simulink model "synth_fir_tb"  (Simulink 7.1)
settings: Solver=ode45  StartTime=0.0  StopTime=160  RelTol=1e-3
undefined symbols (not defined in the file or in its folder): mem
libraries: xbsIndex_r4 x80, xbsCopyrightNotice_r4 x1, dspsigops x1, dspsrcs4 x1
settings Model: Creator=alexc  LastModifiedBy=thuyp
settings DataIOCC: SignalLoggingName=sigsOut
settings OptimizationCC: InlineInvariantSignals=on
settings DebuggingCC: SaveWithParameterizedLinksMsg=none  SignalResolutionControl=TryResolveAllWithWarning  SolverPrmCheckMsg=none  MultiTaskDSMMsg=warning  MultiTaskCondExecSysMsg=none  StrictBusMsg=None
settings HardwareCC: TargetUnknown=on
settings RTWCC: IncludeERTFirstTime=on
settings GRTTargetCC: TargetFcnLib=ansi_tfl_tmw.mat

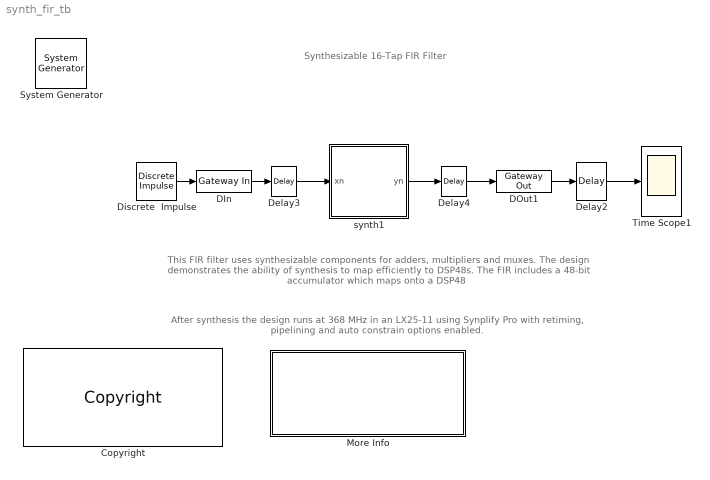
== system synth_fir_tb ==
  note: Synthesizable 16-Tap FIR Filter
  note: This FIR filter uses synthesizable components
      | for adders, multipliers and muxes. The design demonstrates
      |  the ability of synthesis to map efficiently to DSP48s.
      | The FIR includes a 48-bit accumulator which maps onto a DSP48
  note: After synthesis the design runs at 368 MHz in an LX25-11
      | using Synplify Pro with retiming, pipelining and auto constrain options enabled.
  " System Generator" : xbsIndex_r4/ System Generator  Tag=genX  SystemSampleTime=-1  xilinxfamily=virtex4  part=xc4vsx35  speed=-10  package=ff668  synthesis_tool=XST  clock_wrapper=Clock Enables  directory=./netlist  testbench=off  simulink_period=1  sysclk_period=2.90  dcm_input_clock_period=100  incr_netlist=off  trim_vbits=Everywhere in SubSystem  dbl_ovrd=According to Block Masks  core_generation=According to Block Masks  run_coregen=off  deprecated_control=off  eval_field=0  block_type=system_generator
      settings: block_version=8.2.EA1
  Copyright : xbsCopyrightNotice_r4/Copyright  copyrighttext="Copyright (c) 2009  by  Xilinx, Inc. All rights reserved.<br><br>This file contains proprietary, confidential information of Xilinx, Inc., is distributed under licensefrom Xilinx, Inc., and may be used, copied and/or disclosed only pursuant to the terms of a valid licenseagreement with Xilinx, Inc. Xilinx hereby grants you a license to use this file solely for design,simulation, implementation and creation of design files limited to Xilinx devices or technologies. Use with non-Xilinx devices or technologies is expressly prohibited and immediately terminates your license unless covered by a separate agreement.<br><br>Xilinx is providing this design, code, or information \"as-is\" solely for use in developing programs and solutions for Xilinx devices, with no obligation on the part of Xilinx to provide support. By providingthis design, code, or information as one possible implementation of this feature, application or standard,Xilinx is making no representation that this implementation is free from any claims of infringement. Youare responsible for obtaining any rights you may require for your implementation. Xilinx expressly disclaimsany warranty whatsoever with respect to the adequacy of the implementation, including but not limited to anywarranties or representations that this implementation is free from claims of infringement, implied warrantiesof merchantability or fitness for a particular purpose.<br><br>Xilinx products are not intended for use in life support appliances, devices, or systems. Use in such applications is expressly prohibited.<br><br>Any modifications that are made to the Source Code are done at the user's sole risk and will be unsupported.<br><br>This copyright and support notice must be retained as part of this text at all times. (c) Copyright 1995-2009 Xilinx, Inc. All rights reserved."  block_type=copyright
      settings: block_version=10.1.00
      settings: infoedit=|
      | Copyright(C) 2008 by  Xilinx, Inc. All rights reserved.<br>
      | <br>
      | This file contains proprietary, confidential information of Xilinx, Inc., is distributed under license
      | from Xilinx, Inc., and may be used, copied and/or disclosed only pursuant to the terms of a valid license
      | agreement with Xilinx, Inc. Xilinx hereby grants you a license to use this file solely for design,
      | simulation, implementation and creation of design files limited to Xilinx devices or technologies. Use
      | with non-Xilinx devices or technologies is expressly prohibited and immediately terminates your license
      | unless covered by a separate agreement.<br>
      | <br>
      | Xilinx is providing this design, code, or information "as-is" solely for use in developing programs and
      | solutions for Xilinx devices, with no obligation on the part of Xilinx to provide support. By providing
      | this design, code, or information as one possible implementation of this feature, application or standard,
      | Xilinx is making no representation that this implementation is free from any claims of infringement. You
      | are responsible for obtaining any rights you may require for your implementation. Xilinx expressly disclaims
      | any warranty whatsoever with respect to the adequacy of the implementation, including but not limited to any
      | warranties or representations that this implementation is free from claims of infringement, implied warranties
      | of merchantability or fitness for a particular purpose.<br>
      | <br>
      | Xilinx products are not intended for use in life support appliances, devices, or systems. Use in such
      | applications is expressly prohibited.<br>
      | <br>
      | Any modifications that are made to the Source Code are done at the user's sole risk and will be unsupported.<br>
      | <br>
      | This copyright and support notice must be retained as part of this text at all times.
      | (c) Copyright 1995-2008 Xilinx, Inc. All rights reserved.
  DIn : xbsIndex_r4/Gateway In  arith_type="Signed  (2's comp)"  n_bits=18  bin_pt=0  quantization="Round  (unbiased: +/- Inf)"  overflow=Saturate  period=4  dbl_ovrd=off  timing_constraint=None  locs_specified=off  LOCs={}  block_type=gatewayin
      settings: infoedit="Gateway in block.  Converts inputs of type Simulink integer, double and fixed point to  Xilinx fixed point type.<P><P>Hardware notes:  In hardware these blocks become top level input ports."  xl_area=[0 0 0 0 18 0 0]  block_version=VER_STRING_GOES_HERE
  DOut1 : xbsIndex_r4/Gateway Out  hdl_port=on  timing_constraint=None  locs_specified=off  LOCs={}  block_type=gatewayout
      settings: infoedit="Gateway out block.  Converts Xilinx fixed point inputs into ouputs of type Simulink integer, double, or fixed point.<P><P>Hardware notes:  In hardware these blocks become top level output ports or are discarded, depending on how they are configured."  xl_area=[0 0 0 0 48 0 0]  block_version=VER_STRING_GOES_HERE
  Delay2 : dspsigops/Delay  dly_unit=Samples  delay=1  ic_detail=off  dif_ic_for_ch=off  dif_ic_for_dly=off  ic=0  reset_popup=None
  Delay3 : xbsIndex_r4/Delay  en=off  latency=3  dbl_ovrd=off  reg_retiming=on  block_type=delay
      settings: infoedit="Delay line having  configurable length.<P><P>Hardware notes: A delay line is a chain, each link of which is an SRL16 followed by a flip-flop. If register retiming is enabled, the delay line is a chain of flip-flops."  xl_area=[0, 0, 0, 0, 0, 0, 0]  block_version=VER_STRING_GOES_HERE
  Delay4 : xbsIndex_r4/Delay  en=off  latency=3  dbl_ovrd=off  reg_retiming=on  block_type=delay
      settings: infoedit="Delay line having  configurable length.<P><P>Hardware notes: A delay line is a chain, each link of which is an SRL16 followed by a flip-flop. If register retiming is enabled, the delay line is a chain of flip-flops."  xl_area=[0, 0, 0, 0, 0, 0, 0]  block_version=VER_STRING_GOES_HERE
  Discrete  Impulse : dspsrcs4/Discrete  Impulse  Delay=0  SampleTime=4  FrameSample=1  dataType=double  isSigned=on  wordLen=16  udDataType=sfix(16)  fracBitsMode=Best precision  numFracBits=15
  More Info : Subsystem
      settings: OpenFcn=xlDoc('-book','sysgen','-topic','Hardware Design Using System Generator/Design Styles for the DSP48/Designs that Use DSP48 and DSP48 Macro Blocks');
      mask Display: disp('Double click\n for System Generator\n documentation on related topics.')
  Time Scope1 : Scope
      settings: DataFormat=Structure
  synth1 : Subsystem  mask{bit_width=18, bin_pt=0, coef=fir1(15,0.3), coef_bit_width=18, coef_bin_pt=18, m=4, Ts=4}
      mask prompts: bit_width "Input Data Width"; bin_pt "Input Data Binary Point"; coef "Coefficients"; coef_bit_width "Coefficient Bit Width"; coef_bin_pt "Coefficient Binary Point"; m "Number of Multipliers"; Ts "Sample Period"
      mask init:
      | %accounts for the pull down GUI value
      | 
      | no_mults = 4; % for this implementation
      | 
      | %pad the coefficients to be a multiple of the interp_ratio*no_mults
      | multiple_test = ((ceil(length(coef)/no_mults)) - (length(coef)/no_mults)) * no_mults;
      | if (multiple_test > 0)
      | 	coef = [coef(:)' zeros(1,multiple_test)];
      | end
      | 
      | no_taps = length(coef);
      | taps_per_mult = no_taps/no_mults;
      |     
      | %form DRAM values
      | z = zeros(1,taps_per_mult);
      | 
      | for k = 0:(no_mults-1)
      |     for p = 0:(taps_per_mult-1)
      |         mem(p+1,k+1) = coef((k*4)+p+1);
      |     end
      | end
      | 
      | x_SRL_depth = taps_per_mult;
      | upsamp_by = x_SRL_depth;
      | downsamp_by = taps_per_mult;
      | T_clock = Ts/upsamp_by;
      | bit_growth = 2 + ceil(log2(x_SRL_depth));
      | y_bit_width = bit_width + coef_bit_width + bit_growth;
      | 
      | %Display graphic on the block
      | dstr1 = sprintf('%d tap', no_taps);
      | 
      | [bg,fg] = xlcmap('XBlock',0);
      | iPos = get_param(gcb,'Position');
      | iWidth=iPos(3)-iPos(1); iHeight=iPos(4)-iPos(2);
      | iCx=iWidth/2;
      | iCy=iHeight/2;
      | [logoX, logoY] = xlogo(iPos);
      mask StyleString: edit,edit,edit,edit,edit,popup(1|2|3|4|5|6|7|8|9|10|11|12|13|14|15|16|17|18|19|20|21|22|23|24),edit
      mask Display:
      | patch([0 iWidth iWidth 0],[0 0 iHeight iHeight] , bg);
      | patch(logoX,logoY, fg);
      | text(iCx/1.3,iCy+15,dstr1);
      | text(iCx/1.5-4,iCy-5,'MAC FIR');
      | plot([0 0 iWidth iWidth 0], [0 iHeight iHeight 0 0]);
  wires:
  DIn/1 -> Delay3/1
  Discrete  Impulse/1 -> DIn/1
  DOut1/1 -> Delay2/1
  Delay2/1 -> Time Scope1/1
  synth1/1(yn) -> Delay4/1
  Delay3/1 -> synth1/1(xn)
  Delay4/1 -> DOut1/1

== system synth_fir_tb/More Info ==

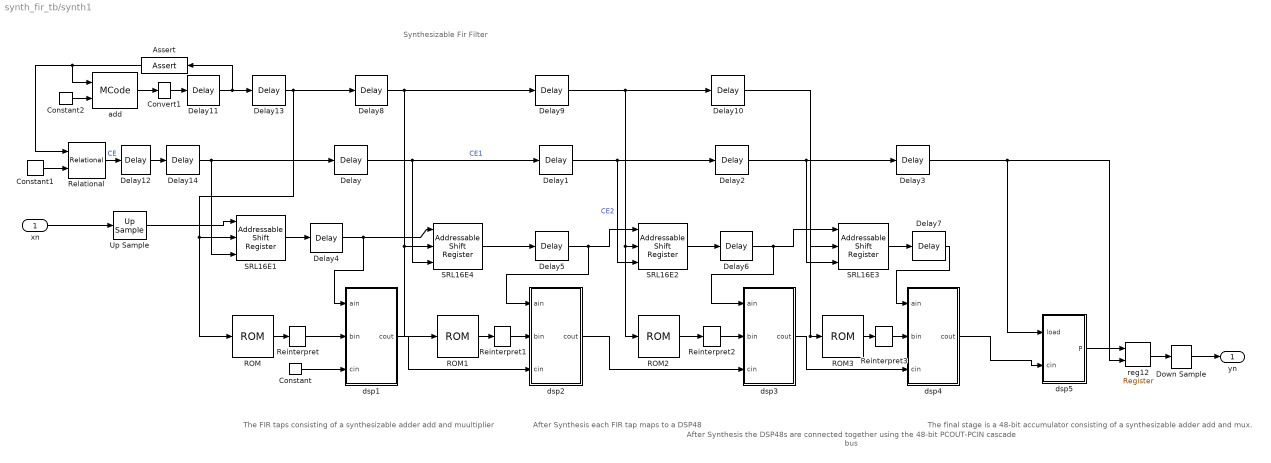
== system synth_fir_tb/synth1 ==
  note: The final stage is a 48-bit accumulator consisting of a
      | synthesizable adder add and mux.
  note: The FIR taps consisting of a
      | synthesizable adder add and muultiplier
  note: After Synthesis each FIR tap maps to a DSP48
  note: After Synthesis the DSP48s are connected together
      | using the 48-bit PCOUT-PCIN cascade bus
  note: Synthesizable Fir Filter
  xn : Inport  OutDataType=sfix(16)  OutScaling=2^0
  Assert : xbsIndex_r4/Assert  Orientation=left  assert_type=off  type_source=Explicitly  arith_type=Unsigned  n_bits=8  bin_pt=2  assert_rate=on  rate_source=Explicitly  period=1  output_port=on  block_type=assert
      settings: infoedit=Asserts a user-defined sample rate and/or type on a signal.  block_version=VER_STRING_GOES_HERE
  Constant : xbsIndex_r4/Constant  arith_type=Signed (2's comp)  const=0  n_bits=48  bin_pt=0  explicit_period=off  period=1  equ=P=C  opselect=C  inp2=PCIN>>17  opr=+  inp1=P  carry=CIN  dbl_ovrd=off  block_type=constant
      settings: block_version=VER_STRING_GOES_HERE
  Constant1 : xbsIndex_r4/Constant  arith_type=Unsigned  const=2  n_bits=2  bin_pt=0  explicit_period=off  period=1  equ=P=C  opselect=C  inp2=PCIN>>17  opr=+  inp1=P  carry=CIN  dbl_ovrd=off  block_type=constant
      settings: block_version=VER_STRING_GOES_HERE
  Constant2 : xbsIndex_r4/Constant  arith_type=Unsigned  const=1  n_bits=2  bin_pt=0  explicit_period=off  period=1  equ=P=C  opselect=C  inp2=PCIN>>17  opr=+  inp1=P  carry=CIN  dbl_ovrd=off  block_type=constant
      settings: block_version=VER_STRING_GOES_HERE
  Convert1 : xbsIndex_r4/Convert  arith_type=Unsigned  n_bits=2  bin_pt=0  quantization=Truncate  overflow=Wrap  latency=0  dbl_ovrd=off  pipeline=off  block_type=convert
      settings: infoedit=The input is presented at the output after quantization and overflow effects.<P><P>Hardware notes: Additional hardware is used when rounding or saturation is selected and output width is less than the input width.  xl_area=[0, 0, 0, 0, 0, 0, 0]  block_version=VER_STRING_GOES_HERE
  Delay{,1..14} (15 alike) : xbsIndex_r4/Delay  en=off  latency=1  dbl_ovrd=off  reg_retiming=on  block_type=delay
      settings: infoedit="Delay line having  configurable length.<P><P>Hardware notes: A delay line is a chain, each link of which is an SRL16 followed by a flip-flop. If register retiming is enabled, the delay line is a chain of flip-flops."  xl_area=[0, 0, 0, 0, 0, 0, 0]  block_version=VER_STRING_GOES_HERE
  Down Sample : xbsIndex_r4/Down Sample  sample_ratio=4  sample_phase="Last Value of Frame  (most efficient)"  en=off  latency=1  dbl_ovrd=off  block_type=dsamp
      settings: xl_area=[24 48 0 0 0 0 0]  block_version=VER_STRING_GOES_HERE
  ROM : xbsIndex_r4/ROM  depth=taps_per_mult  initVector=mem(:,1)  distributed_mem=Distributed memory  rst=off  init_reg=0  en=off  latency=1  arith_type="Signed  (2's comp)"  n_bits=coef_bit_width  bin_pt=coef_bin_pt  dbl_ovrd=off  optimize=Area  use_rpm=off  block_type=sprom
      settings: xl_area=[18 18 0 18 0 0 0]  block_version=VER_STRING_GOES_HERE
  ROM1 : xbsIndex_r4/ROM  depth=taps_per_mult  initVector=mem(:,2)  distributed_mem=Distributed memory  rst=off  init_reg=0  en=off  latency=1  arith_type="Signed  (2's comp)"  n_bits=coef_bit_width  bin_pt=coef_bin_pt  dbl_ovrd=off  optimize=Area  use_rpm=off  block_type=sprom
      settings: xl_area=[18 18 0 17 0 0 0]  block_version=VER_STRING_GOES_HERE
  ROM2 : xbsIndex_r4/ROM  depth=taps_per_mult  initVector=mem(:,3)  distributed_mem=Distributed memory  rst=off  init_reg=0  en=off  latency=1  arith_type="Signed  (2's comp)"  n_bits=coef_bit_width  bin_pt=coef_bin_pt  dbl_ovrd=off  optimize=Area  use_rpm=off  block_type=sprom
      settings: xl_area=[18 18 0 17 0 0 0]  block_version=VER_STRING_GOES_HERE
  ROM3 : xbsIndex_r4/ROM  depth=taps_per_mult  initVector=mem(:,4)  distributed_mem=Distributed memory  rst=off  init_reg=0  en=off  latency=1  arith_type="Signed  (2's comp)"  n_bits=coef_bit_width  bin_pt=coef_bin_pt  dbl_ovrd=off  optimize=Area  use_rpm=off  block_type=sprom
      settings: xl_area=[18 18 0 18 0 0 0]  block_version=VER_STRING_GOES_HERE
  Reinterpret{,1..3} (4 alike) : xbsIndex_r4/Reinterpret  force_arith_type=on  arith_type="Signed  (2's comp)"  force_bin_pt=on  bin_pt=0  block_type=cast
      settings: infoedit="Changes type of samples without altering their binary representation.<P><P>Hardware notes: In hardware this block costs nothing.<P><P>Example:  Suppose the input is 6 bits wide, signed, with 2 fractional bits, and the output is forced to unsigned with 0 fractional bits.  Then an input of -2.0 (1110.00 in binary 2's complement) becomes an output of 56 (111000 in binary)."  block_version=VER_STRING_GOES_HERE
  Relational : xbsIndex_r4/Relational  mode=a=b  en=off  latency=0  dbl_ovrd=off  block_type=relational
      settings: xl_area=[1 0 0 1 0 0 0]  block_version=VER_STRING_GOES_HERE
  SRL16E{1..4} (4 alike) : xbsIndex_r4/Addressable Shift Register  infer_latency=off  depth=x_SRL_depth  initVector=[0]  en=on  dbl_ovrd=off  use_behavioral_HDL=off  use_rpm=off  block_type=addrsr
      settings: infoedit="Delay of configurable length.  Any element in the delay line can be addressed and driven onto the output port.<P><P>Hardware notes: Implemented using SRL16s.  If a Virtex-II device is used, multiple SRLC16s are cascaded together."  xl_area=[9 0 0 18 0 0 0]  block_version=VER_STRING_GOES_HERE
  Up Sample : xbsIndex_r4/Up Sample  sample_ratio=taps_per_mult  copy_samples=on  dbl_ovrd=off  block_type=usamp
      settings: infoedit="Up samples input data.  Inserted values  can be zeros or copies of the most recent input sample.<P><P>Hardware notes: No hardware is needed if inserted values are copies of the input sample; otherwise, a mux and single bit flip-flop are used."  xl_area=[0 0 0 0 0 0 0]  block_version=VER_STRING_GOES_HERE
  add : xbsIndex_r4/MCode  mfname=xlsynadd  explicit_period=off  period=1  dbl_ovrd=off  enable_stdout=off  enable_debug=off  suppress_output=off  defparams={}  hide_port_list={}  block_type=mcode
      settings: xl_area=[0, 0, 0, 0, 0, 0, 0]  block_version=8.1
  dsp1 : Subsystem
  dsp2 : Subsystem
  dsp3 : Subsystem
  dsp4 : Subsystem
  dsp5 : Subsystem
  reg12 : xbsIndex_r4/Register  init=0  rst=off  en=on  dbl_ovrd=off  block_type=register
      settings: xl_area=[24 48 0 0 0 0 0]  block_version=VER_STRING_GOES_HERE
  yn : Outport  OutDataType=sfix(16)  OutScaling=2^0
  wires:
  dsp4/1(cout) -> dsp5/2(cin)
  Convert1/1 -> Delay11/1
  Delay11/1 -> Delay13/1, Assert/1
  add/1 -> Convert1/1
  Constant2/1 -> add/2
  Reinterpret3/1 -> dsp4/2(bin)
  Reinterpret2/1 -> dsp3/2(bin)
  Reinterpret1/1 -> dsp2/2(bin)
  Reinterpret/1 -> dsp1/2(bin)
  ROM/1 -> Reinterpret/1
  Constant/1 -> dsp1/3(cin)
  SRL16E1/1 -> Delay4/1
  SRL16E4/1 -> Delay5/1
  dsp1/1(cout) -> dsp2/3(cin)
  ROM1/1 -> Reinterpret1/1
  ROM2/1 -> Reinterpret2/1
  ROM3/1 -> Reinterpret3/1
  dsp2/1(cout) -> dsp3/3(cin)
  dsp3/1(cout) -> dsp4/3(cin)
  SRL16E2/1 -> Delay6/1
  SRL16E3/1 -> Delay7/1
  Delay10/1 -> SRL16E3/2, ROM3/1
  Delay4/1 -> SRL16E4/1, dsp1/1(ain)
  Delay5/1 -> SRL16E2/1, dsp2/1(ain)
  Delay6/1 -> SRL16E3/1, dsp3/1(ain)
  Constant1/1 -> Relational/2
  Relational/1 -> Delay12/1  "CE"
  Delay2/1 -> Delay3/1, SRL16E3/3
  xn/1 -> Up Sample/1
  dsp5/1(P) -> reg12/1
  Up Sample/1 -> SRL16E1/1
  reg12/1 -> Down Sample/1
  Down Sample/1 -> yn/1
  Delay7/1 -> dsp4/1(ain)
  Delay3/1 -> reg12/2, dsp5/1(load)
  Delay12/1 -> Delay14/1
  Delay8/1 -> Delay9/1, SRL16E4/2, ROM1/1
  Delay9/1 -> Delay10/1, SRL16E2/2, ROM2/1
  Delay1/1 -> Delay2/1, SRL16E2/3  "CE2"
  Delay/1 -> Delay1/1, SRL16E4/3  "CE1"
  Delay13/1 -> Delay8/1, ROM/1, SRL16E1/2
  Delay14/1 -> Delay/1, SRL16E1/3
  Assert/1 -> add/1, Relational/1

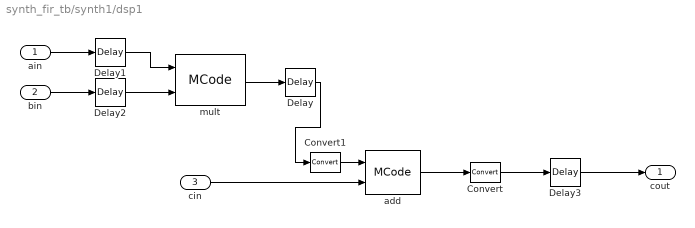
== system synth_fir_tb/synth1/dsp1 ==
  ain : Inport  OutDataType=sfix(16)  OutScaling=2^0
  bin : Inport  Port=2  OutDataType=sfix(16)  OutScaling=2^0
  cin : Inport  Port=3  OutDataType=sfix(16)  OutScaling=2^0
  Convert : xbsIndex_r4/Convert  arith_type="Signed  (2's comp)"  n_bits=48  bin_pt=0  quantization=Truncate  overflow=Wrap  latency=0  dbl_ovrd=off  pipeline=off  block_type=convert
      settings: infoedit=The input is presented at the output after quantization and overflow effects.<P><P>Hardware notes: Additional hardware is used when rounding or saturation is selected and output width is less than the input width.  xl_area=[0, 0, 0, 0, 0, 0, 0]  block_version=VER_STRING_GOES_HERE
  Convert1 : xbsIndex_r4/Convert  arith_type="Signed  (2's comp)"  n_bits=48  bin_pt=0  quantization=Truncate  overflow=Wrap  latency=0  dbl_ovrd=off  pipeline=off  block_type=convert
      settings: infoedit=The input is presented at the output after quantization and overflow effects.<P><P>Hardware notes: Additional hardware is used when rounding or saturation is selected and output width is less than the input width.  xl_area=[0, 0, 0, 0, 0, 0, 0]  block_version=VER_STRING_GOES_HERE
  Delay{,1..3} (4 alike) : xbsIndex_r4/Delay  en=off  latency=1  dbl_ovrd=off  reg_retiming=on  block_type=delay
      settings: infoedit="Delay line having  configurable length.<P><P>Hardware notes: A delay line is a chain, each link of which is an SRL16 followed by a flip-flop. If register retiming is enabled, the delay line is a chain of flip-flops."  xl_area=[0, 0, 0, 0, 0, 0, 0]  block_version=VER_STRING_GOES_HERE
  add : xbsIndex_r4/MCode  mfname=xlsynadd  explicit_period=off  period=1  dbl_ovrd=off  enable_stdout=off  enable_debug=off  suppress_output=off  defparams={}  hide_port_list={}  block_type=mcode
      settings: xl_area=[0, 0, 0, 0, 0, 0, 0]  block_version=8.1
  mult : xbsIndex_r4/MCode  mfname=xlsynmult  explicit_period=off  period=1  dbl_ovrd=off  enable_stdout=off  enable_debug=off  suppress_output=off  defparams={}  hide_port_list={}  block_type=mcode
      settings: xl_area=[0, 0, 0, 0, 0, 0, 0]  block_version=8.1
  cout : Outport  OutDataType=sfix(16)  OutScaling=2^0
  wires:
  Convert1/1 -> add/1
  Convert/1 -> Delay3/1
  Delay/1 -> Convert1/1
  Delay1/1 -> mult/1
  Delay2/1 -> mult/2
  Delay3/1 -> cout/1
  add/1 -> Convert/1
  cin/1 -> add/2
  mult/1 -> Delay/1
  bin/1 -> Delay2/1
  ain/1 -> Delay1/1

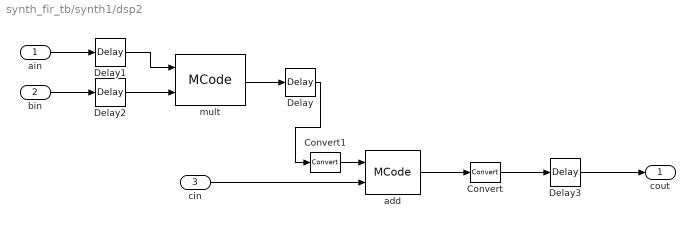
== system synth_fir_tb/synth1/dsp2 ==
  ain : Inport  OutDataType=sfix(16)  OutScaling=2^0
  bin : Inport  Port=2  OutDataType=sfix(16)  OutScaling=2^0
  cin : Inport  Port=3  OutDataType=sfix(16)  OutScaling=2^0
  Convert : xbsIndex_r4/Convert  arith_type="Signed  (2's comp)"  n_bits=48  bin_pt=0  quantization=Truncate  overflow=Wrap  latency=0  dbl_ovrd=off  pipeline=off  block_type=convert
      settings: infoedit=The input is presented at the output after quantization and overflow effects.<P><P>Hardware notes: Additional hardware is used when rounding or saturation is selected and output width is less than the input width.  xl_area=[0, 0, 0, 0, 0, 0, 0]  block_version=VER_STRING_GOES_HERE
  Convert1 : xbsIndex_r4/Convert  arith_type="Signed  (2's comp)"  n_bits=48  bin_pt=0  quantization=Truncate  overflow=Wrap  latency=0  dbl_ovrd=off  pipeline=off  block_type=convert
      settings: infoedit=The input is presented at the output after quantization and overflow effects.<P><P>Hardware notes: Additional hardware is used when rounding or saturation is selected and output width is less than the input width.  xl_area=[0, 0, 0, 0, 0, 0, 0]  block_version=VER_STRING_GOES_HERE
  Delay{,1..3} (4 alike) : xbsIndex_r4/Delay  en=off  latency=1  dbl_ovrd=off  reg_retiming=on  block_type=delay
      settings: infoedit="Delay line having  configurable length.<P><P>Hardware notes: A delay line is a chain, each link of which is an SRL16 followed by a flip-flop. If register retiming is enabled, the delay line is a chain of flip-flops."  xl_area=[0, 0, 0, 0, 0, 0, 0]  block_version=VER_STRING_GOES_HERE
  add : xbsIndex_r4/MCode  mfname=xlsynadd  explicit_period=off  period=1  dbl_ovrd=off  enable_stdout=off  enable_debug=off  suppress_output=off  defparams={}  hide_port_list={}  block_type=mcode
      settings: xl_area=[0, 0, 0, 0, 0, 0, 0]  block_version=8.1
  mult : xbsIndex_r4/MCode  mfname=xlsynmult  explicit_period=off  period=1  dbl_ovrd=off  enable_stdout=off  enable_debug=off  suppress_output=off  defparams={}  hide_port_list={}  block_type=mcode
      settings: xl_area=[0, 0, 0, 0, 0, 0, 0]  block_version=8.1
  cout : Outport  OutDataType=sfix(16)  OutScaling=2^0
  wires:
  ain/1 -> Delay1/1
  bin/1 -> Delay2/1
  mult/1 -> Delay/1
  cin/1 -> add/2
  add/1 -> Convert/1
  Delay3/1 -> cout/1
  Delay2/1 -> mult/2
  Delay1/1 -> mult/1
  Delay/1 -> Convert1/1
  Convert/1 -> Delay3/1
  Convert1/1 -> add/1

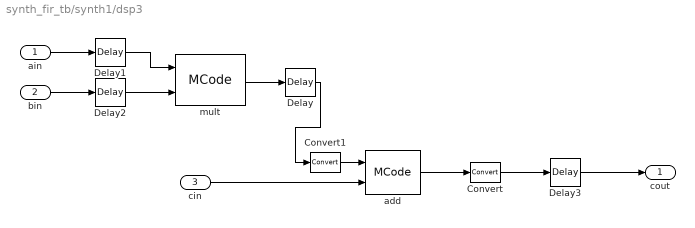
== system synth_fir_tb/synth1/dsp3 ==
  ain : Inport  OutDataType=sfix(16)  OutScaling=2^0
  bin : Inport  Port=2  OutDataType=sfix(16)  OutScaling=2^0
  cin : Inport  Port=3  OutDataType=sfix(16)  OutScaling=2^0
  Convert : xbsIndex_r4/Convert  arith_type="Signed  (2's comp)"  n_bits=48  bin_pt=0  quantization=Truncate  overflow=Wrap  latency=0  dbl_ovrd=off  pipeline=off  block_type=convert
      settings: infoedit=The input is presented at the output after quantization and overflow effects.<P><P>Hardware notes: Additional hardware is used when rounding or saturation is selected and output width is less than the input width.  xl_area=[0, 0, 0, 0, 0, 0, 0]  block_version=VER_STRING_GOES_HERE
  Convert1 : xbsIndex_r4/Convert  arith_type="Signed  (2's comp)"  n_bits=48  bin_pt=0  quantization=Truncate  overflow=Wrap  latency=0  dbl_ovrd=off  pipeline=off  block_type=convert
      settings: infoedit=The input is presented at the output after quantization and overflow effects.<P><P>Hardware notes: Additional hardware is used when rounding or saturation is selected and output width is less than the input width.  xl_area=[0, 0, 0, 0, 0, 0, 0]  block_version=VER_STRING_GOES_HERE
  Delay{,1..3} (4 alike) : xbsIndex_r4/Delay  en=off  latency=1  dbl_ovrd=off  reg_retiming=on  block_type=delay
      settings: infoedit="Delay line having  configurable length.<P><P>Hardware notes: A delay line is a chain, each link of which is an SRL16 followed by a flip-flop. If register retiming is enabled, the delay line is a chain of flip-flops."  xl_area=[0, 0, 0, 0, 0, 0, 0]  block_version=VER_STRING_GOES_HERE
  add : xbsIndex_r4/MCode  mfname=xlsynadd  explicit_period=off  period=1  dbl_ovrd=off  enable_stdout=off  enable_debug=off  suppress_output=off  defparams={}  hide_port_list={}  block_type=mcode
      settings: xl_area=[0, 0, 0, 0, 0, 0, 0]  block_version=8.1
  mult : xbsIndex_r4/MCode  mfname=xlsynmult  explicit_period=off  period=1  dbl_ovrd=off  enable_stdout=off  enable_debug=off  suppress_output=off  defparams={}  hide_port_list={}  block_type=mcode
      settings: xl_area=[0, 0, 0, 0, 0, 0, 0]  block_version=8.1
  cout : Outport  OutDataType=sfix(16)  OutScaling=2^0
  wires:
  Convert1/1 -> add/1
  Convert/1 -> Delay3/1
  Delay/1 -> Convert1/1
  Delay1/1 -> mult/1
  Delay2/1 -> mult/2
  Delay3/1 -> cout/1
  add/1 -> Convert/1
  cin/1 -> add/2
  mult/1 -> Delay/1
  bin/1 -> Delay2/1
  ain/1 -> Delay1/1

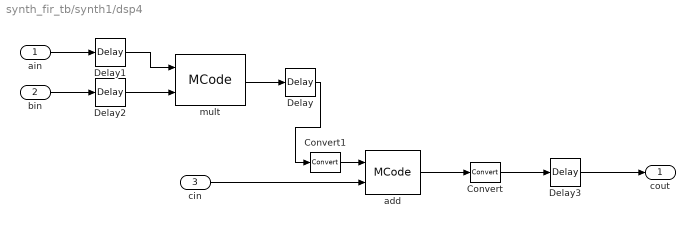
== system synth_fir_tb/synth1/dsp4 ==
  ain : Inport  OutDataType=sfix(16)  OutScaling=2^0
  bin : Inport  Port=2  OutDataType=sfix(16)  OutScaling=2^0
  cin : Inport  Port=3  OutDataType=sfix(16)  OutScaling=2^0
  Convert : xbsIndex_r4/Convert  arith_type="Signed  (2's comp)"  n_bits=48  bin_pt=0  quantization=Truncate  overflow=Wrap  latency=0  dbl_ovrd=off  pipeline=off  block_type=convert
      settings: infoedit=The input is presented at the output after quantization and overflow effects.<P><P>Hardware notes: Additional hardware is used when rounding or saturation is selected and output width is less than the input width.  xl_area=[0, 0, 0, 0, 0, 0, 0]  block_version=VER_STRING_GOES_HERE
  Convert1 : xbsIndex_r4/Convert  arith_type="Signed  (2's comp)"  n_bits=48  bin_pt=0  quantization=Truncate  overflow=Wrap  latency=0  dbl_ovrd=off  pipeline=off  block_type=convert
      settings: infoedit=The input is presented at the output after quantization and overflow effects.<P><P>Hardware notes: Additional hardware is used when rounding or saturation is selected and output width is less than the input width.  xl_area=[0, 0, 0, 0, 0, 0, 0]  block_version=VER_STRING_GOES_HERE
  Delay{,1..3} (4 alike) : xbsIndex_r4/Delay  en=off  latency=1  dbl_ovrd=off  reg_retiming=on  block_type=delay
      settings: infoedit="Delay line having  configurable length.<P><P>Hardware notes: A delay line is a chain, each link of which is an SRL16 followed by a flip-flop. If register retiming is enabled, the delay line is a chain of flip-flops."  xl_area=[0, 0, 0, 0, 0, 0, 0]  block_version=VER_STRING_GOES_HERE
  add : xbsIndex_r4/MCode  mfname=xlsynadd  explicit_period=off  period=1  dbl_ovrd=off  enable_stdout=off  enable_debug=off  suppress_output=off  defparams={}  hide_port_list={}  block_type=mcode
      settings: xl_area=[0, 0, 0, 0, 0, 0, 0]  block_version=8.1
  mult : xbsIndex_r4/MCode  mfname=xlsynmult  explicit_period=off  period=1  dbl_ovrd=off  enable_stdout=off  enable_debug=off  suppress_output=off  defparams={}  hide_port_list={}  block_type=mcode
      settings: xl_area=[0, 0, 0, 0, 0, 0, 0]  block_version=8.1
  cout : Outport  OutDataType=sfix(16)  OutScaling=2^0
  wires:
  ain/1 -> Delay1/1
  bin/1 -> Delay2/1
  mult/1 -> Delay/1
  cin/1 -> add/2
  add/1 -> Convert/1
  Delay3/1 -> cout/1
  Delay2/1 -> mult/2
  Delay1/1 -> mult/1
  Delay/1 -> Convert1/1
  Convert/1 -> Delay3/1
  Convert1/1 -> add/1

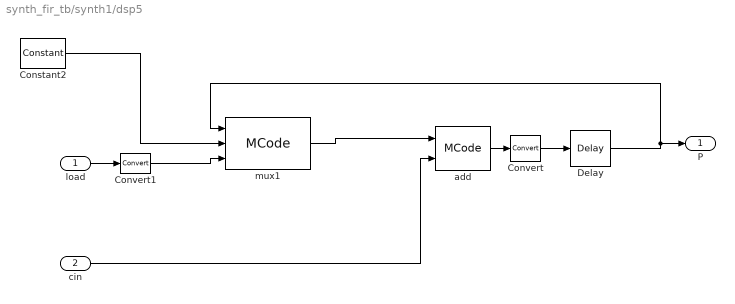
== system synth_fir_tb/synth1/dsp5 ==
  load : Inport  OutDataType=sfix(16)  OutScaling=2^0
  cin : Inport  Port=2  OutDataType=sfix(16)  OutScaling=2^0
  Constant2 : xbsIndex_r4/Constant  arith_type=Signed (2's comp)  const=0  n_bits=48  bin_pt=0  explicit_period=on  period=1  equ=P=C  opselect=C  inp2=PCIN>>17  opr=+  inp1=P  carry=CIN  dbl_ovrd=off  block_type=constant
      settings: block_version=VER_STRING_GOES_HERE
  Convert : xbsIndex_r4/Convert  arith_type="Signed  (2's comp)"  n_bits=48  bin_pt=0  quantization=Truncate  overflow=Wrap  latency=0  dbl_ovrd=off  pipeline=off  block_type=convert
      settings: infoedit=The input is presented at the output after quantization and overflow effects.<P><P>Hardware notes: Additional hardware is used when rounding or saturation is selected and output width is less than the input width.  xl_area=[0, 0, 0, 0, 0, 0, 0]  block_version=VER_STRING_GOES_HERE
  Convert1 : xbsIndex_r4/Convert  arith_type=Unsigned  n_bits=1  bin_pt=0  quantization=Truncate  overflow=Wrap  latency=0  dbl_ovrd=off  pipeline=off  block_type=convert
      settings: infoedit=The input is presented at the output after quantization and overflow effects.<P><P>Hardware notes: Additional hardware is used when rounding or saturation is selected and output width is less than the input width.  xl_area=[0, 0, 0, 0, 0, 0, 0]  block_version=VER_STRING_GOES_HERE
  Delay : xbsIndex_r4/Delay  en=off  latency=1  dbl_ovrd=off  reg_retiming=on  block_type=delay
      settings: infoedit="Delay line having  configurable length.<P><P>Hardware notes: A delay line is a chain, each link of which is an SRL16 followed by a flip-flop. If register retiming is enabled, the delay line is a chain of flip-flops."  xl_area=[0, 0, 0, 0, 0, 0, 0]  block_version=VER_STRING_GOES_HERE
  add : xbsIndex_r4/MCode  mfname=xlsynadd  explicit_period=off  period=1  dbl_ovrd=off  enable_stdout=off  enable_debug=off  suppress_output=off  defparams={}  hide_port_list={}  block_type=mcode
      settings: xl_area=[0, 0, 0, 0, 0, 0, 0]  block_version=8.1
  mux1 : xbsIndex_r4/MCode  mfname=xlsynmux  explicit_period=off  period=1  dbl_ovrd=off  enable_stdout=off  enable_debug=off  suppress_output=off  defparams={}  hide_port_list={}  block_type=mcode
      settings: xl_area=[0, 0, 0, 0, 0, 0, 0]  block_version=8.1
  P : Outport  OutDataType=sfix(16)  OutScaling=2^0
  wires:
  Convert/1 -> Delay/1
  mux1/1 -> add/1
  add/1 -> Convert/1
  Delay/1 -> mux1/1, P/1
  cin/1 -> add/2
  load/1 -> Convert1/1
  Constant2/1 -> mux1/2
  Convert1/1 -> mux1/3
